simulink model "Self_Made_VCO"  (R2019b)
settings: Solver=VariableStepAuto  StartTime=0.0  StopTime=0.00000005  RelTol=1e-3
settings Model: Creator=connerhannon  LastModifiedBy=connerhannon
settings SolverCC: MaxConsecutiveZCs=1  MaxConsecutiveMinStep=100000

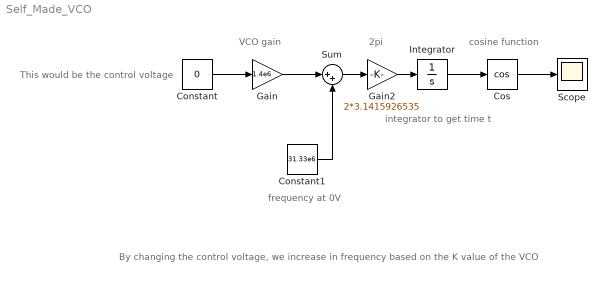
== system Self_Made_VCO ==
  note: By changing the control voltage, we increase in frequency based on the K value of the VCO
  note: cosine function
  note: integrator to get time t
  note: 2pi
  note: frequency at 0V
  note: VCO gain
  note: This would be the control voltage
  Constant : Constant  Value=0
  Constant1 : Constant  Value=31.33e6
  Cos : Trigonometry  Operator=cos
  Gain : Gain  Gain=1.4e6
  Gain2 : Gain  Gain=2*3.1415926535
  Integrator : Integrator
  Scope : Scope
  Sum : Sum  Inputs=|++
  wires:
  Gain/1 -> Sum/1
  Constant1/1 -> Sum/2
  Constant/1 -> Gain/1
  Sum/1 -> Gain2/1
  Gain2/1 -> Integrator/1
  Integrator/1 -> Cos/1
  Cos/1 -> Scope/1
